simulink model "external_memory_test"  (R2020b)
settings: Solver=FixedStepDiscrete  StartTime=0.0  StopTime=80  RelTol=1e-3
InitFcn:
  | Feature_Width = 64;
  | Feature_Height = 64;
  | Weight_Width = 3;
  | Weight_Height = 3;
  | external_memory_test_init;
values from neighbouring files (symbols this model uses):
  Burst_Length = Feature_Weight_Length    [external_memory_test_init.m]
  byPass = 1    [external_memory_test_init.m]
  Conv_Padding = 0    [external_memory_test_init.m]
  Conv_Stride = 1    [external_memory_test_init.m]
  DDR_Depth = Weight_Length + Feature_Length + outFeature_Length    [external_memory_test_init.m]
  ddrInitData = single((rand(1,DDR_Depth)))    [external_memory_test_init.m]
  Duty_Cycle = 0.5    [external_memory_test_init.m]
  Feature_Area = Feature_Width * Feature_Height    [external_memory_test_init.m]
  Feature_Length = Phase_In * Feature_Area    [external_memory_test_init.m]
  inChannel = 3    [external_memory_test_init.m]
  outChannel = 2    [external_memory_test_init.m]
  outFeature_Length = outFeature_Width * outFeature_Height * Phase_Out    [external_memory_test_init.m]
  Pool_Stride = 2    [external_memory_test_init.m]
  Pool_Width = 2    [external_memory_test_init.m]
  Tc = 1    [external_memory_test_init.m]
  Ti = 1    [external_memory_test_init.m]
  To = 1    [external_memory_test_init.m]
  Tr = 1    [external_memory_test_init.m]
  Weight_Length = Phase_In * Weight_Area * Phase_Out    [external_memory_test_init.m]
undefined symbols (not defined in the file or in its folder): Conv_Step, Pool_Step, sigbuilder_block
libraries: hdlsllib x85, simulink x44, visionhdlutilities x16
(part 3 of 6)

== system external_memory_test/DUT/2DConvPE V1.0/Subsystem2 ==
  In1 : Inport
  Bus Selector : BusSelector  OutputSignals=signal1,signal2,signal3,signal4,signal5,signal6,signal7,signal8,signal9,signal10,signal11,signal12,signal13,signal14,signal15
  Weight_Length : Outport
  Weight_Area : Outport  Port=2
  Weight_Width : Outport  Port=3
  Weight_Height : Outport  Port=4
  Feature_Length : Outport  Port=5
  Feature_Area : Outport  Port=6
  Feature_Width : Outport  Port=7
  Feature_Height : Outport  Port=8
  outFeature_Length : Outport  Port=9
  outFeature_Area : Outport  Port=10
  outFeature_Width : Outport  Port=11
  outFeature_Height : Outport  Port=12
  Conv_Step : Outport  Port=13
  inChannel : Outport  Port=14
  outChannel : Outport  Port=15
  wires:
  In1/1 -> Bus Selector/1
  Bus Selector/1 -> Weight_Length/1  "<signal1>"
  Bus Selector/2 -> Weight_Area/1  "<signal2>"
  Bus Selector/3 -> Weight_Width/1  "<signal3>"
  Bus Selector/4 -> Weight_Height/1  "<signal4>"
  Bus Selector/5 -> Feature_Length/1  "<signal5>"
  Bus Selector/6 -> Feature_Area/1  "<signal6>"
  Bus Selector/7 -> Feature_Width/1  "<signal7>"
  Bus Selector/8 -> Feature_Height/1  "<signal8>"
  Bus Selector/9 -> outFeature_Length/1  "<signal9>"
  Bus Selector/10 -> outFeature_Area/1  "<signal10>"
  Bus Selector/11 -> outFeature_Width/1  "<signal11>"
  Bus Selector/12 -> outFeature_Height/1  "<signal12>"
  Bus Selector/13 -> Conv_Step/1  "<signal13>"
  Bus Selector/14 -> inChannel/1  "<signal14>"
  Bus Selector/15 -> outChannel/1  "<signal15>"

== system external_memory_test/DUT/2DConvPE V1.0/Window Selector ==
  In1 : Inport
  valid : Inport  Port=2
  step : Inport  Port=3
  Add : Sum  Inputs=+-
  Compare To Zero : simulink/Logic and Bit Operations/Compare To Zero  relop===  OutDataTypeStr=boolean
  Constant : Constant  OutDataTypeStr=uint32
  Delay : Delay
  Delay1 : Delay  DelayLength=3
  Delay2 : Delay  DelayLength=1
  Delay3 : Delay  DelayLength=1
  Delay4 : Delay  DelayLength=1
  Logical Operator : Logic  Operator=NOT  AllPortsSameDT=off  OutDataTypeStr=boolean
  Logical Operator1 : Logic  Operator=OR  AllPortsSameDT=off  OutDataTypeStr=boolean
  Logical Operator2 : Logic  AllPortsSameDT=off  OutDataTypeStr=boolean
  Relational Operator : RelationalOperator  OutDataTypeStr=boolean  RndMeth=Nearest
  Selector1 : Selector  InputPortWidth=3  IndexOptions=Index vector (dialog)  Indices=[1]  OutputSizes=1
  Selector2 : Selector  InputPortWidth=3  IndexOptions=Index vector (dialog)  Indices=[2]  OutputSizes=1
  Selector3 : Selector  InputPortWidth=3  IndexOptions=Index vector (dialog)  Indices=[3]  OutputSizes=1
  Selector4 : Selector  InputPortWidth=3  IndexOptions=Index vector (dialog)  Indices=[1]  OutputSizes=1
  Selector5 : Selector  InputPortWidth=3  IndexOptions=Index vector (dialog)  Indices=[2]  OutputSizes=1
  Selector6 : Selector  InputPortWidth=3  IndexOptions=Index vector (dialog)  Indices=[3]  OutputSizes=1
  Selector7 : Selector  InputPortWidth=3  IndexOptions=Index vector (dialog)  Indices=[1]  OutputSizes=1
  Selector8 : Selector  InputPortWidth=3  IndexOptions=Index vector (dialog)  Indices=[2]  OutputSizes=1
  Selector9 : Selector  InputPortWidth=3  IndexOptions=Index vector (dialog)  Indices=[3]  OutputSizes=1
  Step Counter : hdlsllib/Sources/HDL Counter  CountType=Free running  CountInit=0  CountStep=1  CountMax=2^15  CountFromType=Initial value  CountFrom=0  CountResetPort=on  CountLoadPort=off  CountEnbPort=on  CountDirPort=off  CountDataType=Unsigned  CountWordLen=32  CountFracLen=0  CountSampTime=1
  Out1 : Outport
  Out2 : Outport  Port=2
  Out3 : Outport  Port=3
  Out4 : Outport  Port=4
  Out5 : Outport  Port=5
  Out6 : Outport  Port=6
  Out7 : Outport  Port=7
  Out8 : Outport  Port=8
  Out9 : Outport  Port=9
  Valid : Outport  Port=10
  wires:
  Selector2/1 -> Out2/1
  In1/1 -> Delay2/1, Delay1/1, Delay/1
  Selector1/1 -> Out1/1
  Selector3/1 -> Out3/1
  Selector8/1 -> Out5/1
  Selector9/1 -> Out6/1
  Selector7/1 -> Out4/1
  Delay/1 -> Selector9/1, Selector8/1, Selector7/1
  Selector5/1 -> Out8/1
  Selector6/1 -> Out9/1
  Selector4/1 -> Out7/1
  Delay1/1 -> Selector6/1, Selector5/1, Selector4/1
  Relational Operator/1 -> Logical Operator1/1
  Constant/1 -> Add/2
  Logical Operator2/1 -> Valid/1
  Compare To Zero/1 -> Logical Operator2/1
  Logical Operator1/1 -> Step Counter/1
  Logical Operator/1 -> Logical Operator1/2
  Delay4/1 -> Add/1
  Step Counter/1 -> Compare To Zero/1, Relational Operator/1
  Delay3/1 -> Logical Operator2/2, Step Counter/2, Logical Operator/1
  Add/1 -> Relational Operator/2
  Delay2/1 -> Selector3/1, Selector2/1, Selector1/1
  valid/1 -> Delay3/1
  step/1 -> Delay4/1

== system external_memory_test/DUT/2DConvPE V1.1/Adder Tree ==
  In1 : Inport
  In2 : Inport  Port=2
  In3 : Inport  Port=3
  In4 : Inport  Port=4
  In5 : Inport  Port=5
  In6 : Inport  Port=6
  In7 : Inport  Port=7
  In8 : Inport  Port=8
  In9 : Inport  Port=9
  validIn : Inport  Port=10
  Add{,1..6,10} (8 alike) : Sum
  Delay{1..9,35} (10 alike) : Delay  DelayLength=1
  Out1 : Outport
  validOut : Outport  Port=2
  wires:
  Add/1 -> Add4/1
  Add4/1 -> Add6/1
  Add10/1 -> Out1/1
  Add3/1 -> Add5/2
  Add2/1 -> Add5/1
  Add1/1 -> Add4/2
  Add6/1 -> Add10/1
  Add5/1 -> Add6/2
  Delay35/1 -> Add/1
  Delay1/1 -> Add/2
  Delay3/1 -> Add1/1
  Delay2/1 -> Add1/2
  Delay5/1 -> Add2/1
  Delay4/1 -> Add2/2
  Delay7/1 -> Add3/1
  Delay6/1 -> Add3/2
  In9/1 -> Delay8/1
  Delay8/1 -> Add10/2
  In8/1 -> Delay6/1
  In7/1 -> Delay7/1
  In6/1 -> Delay4/1
  In5/1 -> Delay5/1
  In4/1 -> Delay2/1
  In3/1 -> Delay3/1
  In2/1 -> Delay1/1
  In1/1 -> Delay35/1
  validIn/1 -> Delay9/1
  Delay9/1 -> validOut/1

== system external_memory_test/DUT/2DConvPE V1.1/Address Logic ==
  note: W/R_Address_Gen
  In1 : Inport
  In2 : Inport  Port=2
  " " : Subsystem
  Add : Sum  Inputs=+-
  Compare To Constant : simulink/Logic and Bit Operations/Compare To Constant  relop===  const=0  OutDataTypeStr=boolean
  Constant : Constant  OutDataTypeStr=uint32
  Delay : Delay  DelayLength=1
  Logical Operator1 : Logic  AllPortsSameDT=off  OutDataTypeStr=boolean
  Logical Operator2 : Logic  Operator=NOT  AllPortsSameDT=off  OutDataTypeStr=boolean
  Relational Operator : RelationalOperator  OutDataTypeStr=boolean  RndMeth=Simplest
  Weight_Counter : hdlsllib/Sources/HDL Counter  CountType=Free running  CountInit=0  CountStep=1  CountMax=2^15  CountFromType=Initial value  CountFrom=0  CountResetPort=on  CountLoadPort=off  CountEnbPort=on  CountDirPort=off  CountDataType=Unsigned  CountWordLen=32  CountFracLen=0  CountSampTime=1
  Weight_Interation_Counter : hdlsllib/Sources/HDL Counter  CountType=Free running  CountInit=0  CountStep=1  CountMax=2^15  CountFromType=Initial value  CountFrom=0  CountResetPort=on  CountLoadPort=off  CountEnbPort=on  CountDirPort=off  CountDataType=Unsigned  CountWordLen=32  CountFracLen=0  CountSampTime=1
  W : Outport
  Write_en : Outport  Port=2
  R : Outport  Port=3
  wires:
  Weight_Counter/1 -> " "/1(In1), Relational Operator/1
  Compare To Constant/1 -> Write_en/1, " "/2(In2)
  Delay/1 -> Logical Operator1/2, Logical Operator2/1, Weight_Counter/2
  Weight_Interation_Counter/1 -> Compare To Constant/1
  Constant/1 -> Add/2
  Logical Operator2/1 -> Weight_Interation_Counter/1
  " "/1(W) -> W/1
  Logical Operator1/1 -> Weight_Counter/1
  Relational Operator/1 -> Weight_Interation_Counter/2, Logical Operator1/1
  Add/1 -> Relational Operator/2
  In1/1 -> Delay/1
  In2/1 -> Add/1
  " "/2(R) -> R/1

== system external_memory_test/DUT/2DConvPE V1.1/AddressGen ==
  enb : Inport
  PhaseOut_Count : Inport  Port=2
  outFeature_Area : Inport  Port=3
  ADD : Sum
  Constant1 : Constant  Value=0  OutDataTypeStr=uint32  SampleTime=-1
  Constant2 : Constant  OutDataTypeStr=uint32  SampleTime=-1
  Minus : Sum  Inputs=+-
  OutAddress_Counter : hdlsllib/Sources/HDL Counter  CountType=Free running  CountInit=0  CountStep=1  CountMax=2^15  CountFromType=Initial value  CountFrom=0  CountResetPort=on  CountLoadPort=off  CountEnbPort=on  CountDirPort=off  CountDataType=Unsigned  CountWordLen=32  CountFracLen=0  CountSampTime=1
  Product : Product
  Relational Operator : RelationalOperator  OutDataTypeStr=boolean  RndMeth=Nearest
  Switch : Switch  Criteria=u2 ~= 0
  OutAdddess : Outport
  wires:
  Constant1/1 -> Switch/1
  Switch/1 -> Product/2
  OutAddress_Counter/1 -> Relational Operator/1, ADD/2
  outFeature_Area/1 -> Product/1, Minus/1
  Relational Operator/1 -> OutAddress_Counter/1
  Constant2/1 -> Minus/2
  Product/1 -> ADD/1
  ADD/1 -> OutAdddess/1
  Minus/1 -> Relational Operator/2
  enb/1 -> Switch/2, OutAddress_Counter/2
  PhaseOut_Count/1 -> Switch/3

== system external_memory_test/DUT/2DConvPE V1.1/LIne Buffer ==
  Stream_In : Inport
  Stream_Valid : Inport  Port=2
  Weight_Width : Inport  Port=3
  Feature_Area : Inport  Port=4
  Feature_Width : Inport  Port=5
  Feature_Height : Inport  Port=6
  Delay2 : Delay  DelayLength=1
  Line Buffer : Subsystem
  OutValidGen : Subsystem
  Terminator : Terminator
  pixel : Outport
  valid : Outport  Port=2
  wires:
  Feature_Area/1 -> Line Buffer/3(Feature_Area)
  Feature_Height/1 -> OutValidGen/3(Feature_Height)
  Line Buffer/3(shftEnable) -> Terminator/1
  Stream_In/1 -> Line Buffer/1(Stream_In)
  Line Buffer/1(pixel) -> Delay2/1
  Line Buffer/2(ctrl) -> OutValidGen/1(In1)
  Feature_Width/1 -> Line Buffer/4(Feature_Width)
  Stream_Valid/1 -> Line Buffer/2(Stream_Valid)
  Weight_Width/1 -> OutValidGen/2(Weight_Width)
  OutValidGen/1(valid) -> valid/1
  Delay2/1 -> pixel/1

== system external_memory_test/DUT/2DConvPE V1.1/MaxPooling ==
  Stream_In : Inport
  Stream_Valid : Inport  Port=2
  ByPass : Inport  Port=3
  step : Inport  Port=4
  Window_Width : Inport  Port=5
  Feature_Area : Inport  Port=6
  Feature_Width : Inport  Port=7
  Feature_Height : Inport  Port=8
  Comparator : Subsystem
  Constant : Constant  Value=0  OutDataTypeStr=int32
  Delay{,1..6,36} (8 alike) : Delay  DelayLength=1
  Line Buffer1 : Subsystem
  OutValidGen : Subsystem
  Switch : Switch  Criteria=u2 > Threshold
  Switch1 : Switch  Criteria=u2 > Threshold
  Terminator1 : Terminator
  dataSwitch : Switch  Criteria=u2 > Threshold
  validSwitch : Switch  Criteria=u2 > Threshold
  window Selector : Subsystem
  outdata : Outport
  Valid : Outport  Port=2
  wires:
  window Selector/3(Out3) -> Delay3/1
  OutValidGen/1(Out1) -> window Selector/2(valid)
  Feature_Width/1 -> Line Buffer1/4(Feature_Width)
  Line Buffer1/3(shftEnable) -> Terminator1/1
  Window_Width/1 -> OutValidGen/2(Window_Width)
  window Selector/5(Valid) -> Delay5/1
  window Selector/1(Out1) -> Delay/1
  Line Buffer1/1(pixel) -> Delay2/1
  Line Buffer1/2(ctrl) -> OutValidGen/1(ctrl)
  window Selector/2(Out2) -> Delay6/1
  window Selector/4(Out4) -> Delay4/1
  Feature_Area/1 -> Line Buffer1/3(Feature_Area)
  Feature_Height/1 -> OutValidGen/3(Feature_Height)
  step/1 -> window Selector/3(step)
  Delay1/1 -> validSwitch/1, Switch1/3
  Comparator/1(Out1) -> dataSwitch/3
  Delay36/1 -> dataSwitch/1, Switch/3
  ByPass/1 -> validSwitch/2, dataSwitch/2, Switch1/2, Switch/2
  dataSwitch/1 -> outdata/1
  validSwitch/1 -> Valid/1
  Constant/1 -> Switch1/1, Switch/1
  Switch/1 -> Line Buffer1/1(Stream_In)
  Switch1/1 -> Line Buffer1/2(Stream_Valid)
  Comparator/2(outvalid) -> validSwitch/3
  Stream_In/1 -> Delay36/1
  Stream_Valid/1 -> Delay1/1
  Delay2/1 -> window Selector/1(pixel)
  Delay/1 -> Comparator/1(In1)
  Delay5/1 -> Comparator/5(Valid)
  Delay4/1 -> Comparator/4(In4)
  Delay3/1 -> Comparator/3(In3)
  Delay6/1 -> Comparator/2(In2)

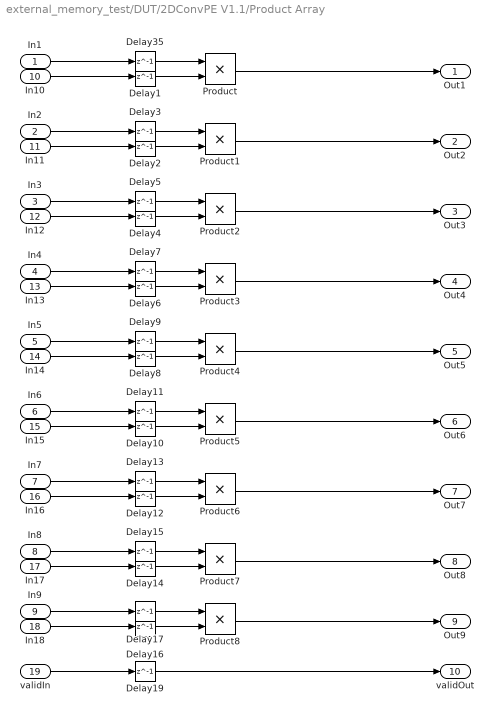
== system external_memory_test/DUT/2DConvPE V1.1/Product Array ==
  In1 : Inport
  In2 : Inport  Port=2
  In3 : Inport  Port=3
  In4 : Inport  Port=4
  In5 : Inport  Port=5
  In6 : Inport  Port=6
  In7 : Inport  Port=7
  In8 : Inport  Port=8
  In9 : Inport  Port=9
  In10 : Inport  Port=10
  In11 : Inport  Port=11
  In12 : Inport  Port=12
  In13 : Inport  Port=13
  In14 : Inport  Port=14
  In15 : Inport  Port=15
  In16 : Inport  Port=16
  In17 : Inport  Port=17
  In18 : Inport  Port=18
  validIn : Inport  Port=19
  Delay{1..17,19,35} (19 alike) : Delay  DelayLength=1
  Product{,1..8} (9 alike) : Product
  Out1 : Outport
  Out2 : Outport  Port=2
  Out3 : Outport  Port=3
  Out4 : Outport  Port=4
  Out5 : Outport  Port=5
  Out6 : Outport  Port=6
  Out7 : Outport  Port=7
  Out8 : Outport  Port=8
  Out9 : Outport  Port=9
  validOut : Outport  Port=10
  wires:
  Product/1 -> Out1/1
  In4/1 -> Delay7/1
  Product4/1 -> Out5/1
  In8/1 -> Delay15/1
  In17/1 -> Delay14/1
  In9/1 -> Delay17/1
  In12/1 -> Delay4/1
  In7/1 -> Delay13/1
  In1/1 -> Delay35/1
  In13/1 -> Delay6/1
  Product1/1 -> Out2/1
  In16/1 -> Delay12/1
  In10/1 -> Delay1/1
  In14/1 -> Delay8/1
  In18/1 -> Delay16/1
  Product8/1 -> Out9/1
  Product7/1 -> Out8/1
  In6/1 -> Delay11/1
  In2/1 -> Delay3/1
  In11/1 -> Delay2/1
  In15/1 -> Delay10/1
  In5/1 -> Delay9/1
  In3/1 -> Delay5/1
  Product3/1 -> Out4/1
  Product2/1 -> Out3/1
  Product5/1 -> Out6/1
  Product6/1 -> Out7/1
  validIn/1 -> Delay19/1
  Delay1/1 -> Product/2
  Delay35/1 -> Product/1
  Delay3/1 -> Product1/1
  Delay2/1 -> Product1/2
  Delay5/1 -> Product2/1
  Delay4/1 -> Product2/2
  Delay7/1 -> Product3/1
  Delay6/1 -> Product3/2
  Delay8/1 -> Product4/2
  Delay9/1 -> Product4/1
  Delay11/1 -> Product5/1
  Delay10/1 -> Product5/2
  Delay13/1 -> Product6/1
  Delay12/1 -> Product6/2
  Delay14/1 -> Product7/2
  Delay15/1 -> Product7/1
  Delay17/1 -> Product8/1
  Delay16/1 -> Product8/2
  Delay19/1 -> validOut/1

== system external_memory_test/DUT/2DConvPE V1.1/ReLU ==
  data_in : Inport
  validIn : Inport  Port=2
  byPass : Inport  Port=3
  Compare To Zero : simulink/Logic and Bit Operations/Compare To Zero  relop=>  OutDataTypeStr=boolean
  Constant : Constant  Value=0  OutDataTypeStr=int32
  Delay1 : Delay  DelayLength=1
  Delay36 : Delay  DelayLength=1
  Switch : Switch  Criteria=u2 > Threshold
  Switch1 : Switch  Criteria=u2 > Threshold
  data_ReLU : Outport
  valildOut : Outport  Port=2
  wires:
  Constant/1 -> Switch/3
  Delay36/1 -> Switch1/1, Switch/1, Compare To Zero/1
  Compare To Zero/1 -> Switch/2
  Switch/1 -> Switch1/3
  byPass/1 -> Switch1/2
  Switch1/1 -> data_ReLU/1
  Delay1/1 -> valildOut/1
  data_in/1 -> Delay36/1
  validIn/1 -> Delay1/1

== system external_memory_test/DUT/2DConvPE V1.1/Subsystem ==
  In1 : Inport
  Bus Selector : BusSelector  OutputSignals=signal1,signal2
  pool_step : Outport
  pool_Width : Outport  Port=2
  wires:
  Bus Selector/2 -> pool_Width/1  "<signal2>"
  Bus Selector/1 -> pool_step/1  "<signal1>"
  In1/1 -> Bus Selector/1

== system external_memory_test/DUT/2DConvPE V1.1/Subsystem2 ==
  In1 : Inport
  Bus Selector : BusSelector  OutputSignals=signal1,signal2,signal3,signal4,signal5,signal6,signal7,signal8,signal9,signal10,signal11,signal12,signal13,signal14,signal15
  Weight_Length : Outport
  Weight_Area : Outport  Port=2
  Weight_Width : Outport  Port=3
  Weight_Height : Outport  Port=4
  Feature_Length : Outport  Port=5
  Feature_Area : Outport  Port=6
  Feature_Width : Outport  Port=7
  Feature_Height : Outport  Port=8
  outFeature_Length : Outport  Port=9
  outFeature_Area : Outport  Port=10
  outFeature_Width : Outport  Port=11
  outFeature_Height : Outport  Port=12
  Conv_Step : Outport  Port=13
  inChannel : Outport  Port=14
  outChannel : Outport  Port=15
  wires:
  In1/1 -> Bus Selector/1
  Bus Selector/1 -> Weight_Length/1  "<signal1>"
  Bus Selector/2 -> Weight_Area/1  "<signal2>"
  Bus Selector/3 -> Weight_Width/1  "<signal3>"
  Bus Selector/4 -> Weight_Height/1  "<signal4>"
  Bus Selector/5 -> Feature_Length/1  "<signal5>"
  Bus Selector/6 -> Feature_Area/1  "<signal6>"
  Bus Selector/7 -> Feature_Width/1  "<signal7>"
  Bus Selector/8 -> Feature_Height/1  "<signal8>"
  Bus Selector/9 -> outFeature_Length/1  "<signal9>"
  Bus Selector/10 -> outFeature_Area/1  "<signal10>"
  Bus Selector/11 -> outFeature_Width/1  "<signal11>"
  Bus Selector/12 -> outFeature_Height/1  "<signal12>"
  Bus Selector/13 -> Conv_Step/1  "<signal13>"
  Bus Selector/14 -> inChannel/1  "<signal14>"
  Bus Selector/15 -> outChannel/1  "<signal15>"

== system external_memory_test/DUT/2DConvPE V1.1/Window Selector ==
  In1 : Inport
  valid : Inport  Port=2
  step : Inport  Port=3
  Add : Sum  Inputs=+-
  Compare To Zero : simulink/Logic and Bit Operations/Compare To Zero  relop===  OutDataTypeStr=boolean
  Constant : Constant  OutDataTypeStr=uint32
  Delay : Delay
  Delay1 : Delay  DelayLength=3
  Delay2 : Delay  DelayLength=1
  Delay3 : Delay  DelayLength=1
  Delay4 : Delay  DelayLength=1
  Logical Operator : Logic  Operator=NOT  AllPortsSameDT=off  OutDataTypeStr=boolean
  Logical Operator1 : Logic  Operator=OR  AllPortsSameDT=off  OutDataTypeStr=boolean
  Logical Operator2 : Logic  AllPortsSameDT=off  OutDataTypeStr=boolean
  Relational Operator : RelationalOperator  OutDataTypeStr=boolean  RndMeth=Nearest
  Selector1 : Selector  InputPortWidth=3  IndexOptions=Index vector (dialog)  Indices=[1]  OutputSizes=1
  Selector2 : Selector  InputPortWidth=3  IndexOptions=Index vector (dialog)  Indices=[2]  OutputSizes=1
  Selector3 : Selector  InputPortWidth=3  IndexOptions=Index vector (dialog)  Indices=[3]  OutputSizes=1
  Selector4 : Selector  InputPortWidth=3  IndexOptions=Index vector (dialog)  Indices=[1]  OutputSizes=1
  Selector5 : Selector  InputPortWidth=3  IndexOptions=Index vector (dialog)  Indices=[2]  OutputSizes=1
  Selector6 : Selector  InputPortWidth=3  IndexOptions=Index vector (dialog)  Indices=[3]  OutputSizes=1
  Selector7 : Selector  InputPortWidth=3  IndexOptions=Index vector (dialog)  Indices=[1]  OutputSizes=1
  Selector8 : Selector  InputPortWidth=3  IndexOptions=Index vector (dialog)  Indices=[2]  OutputSizes=1
  Selector9 : Selector  InputPortWidth=3  IndexOptions=Index vector (dialog)  Indices=[3]  OutputSizes=1
  Step Counter : hdlsllib/Sources/HDL Counter  CountType=Free running  CountInit=0  CountStep=1  CountMax=2^15  CountFromType=Initial value  CountFrom=0  CountResetPort=on  CountLoadPort=off  CountEnbPort=on  CountDirPort=off  CountDataType=Unsigned  CountWordLen=32  CountFracLen=0  CountSampTime=1
  Out1 : Outport
  Out2 : Outport  Port=2
  Out3 : Outport  Port=3
  Out4 : Outport  Port=4
  Out5 : Outport  Port=5
  Out6 : Outport  Port=6
  Out7 : Outport  Port=7
  Out8 : Outport  Port=8
  Out9 : Outport  Port=9
  Valid : Outport  Port=10
  wires:
  Selector2/1 -> Out2/1
  In1/1 -> Delay2/1, Delay1/1, Delay/1
  Selector1/1 -> Out1/1
  Selector3/1 -> Out3/1
  Selector8/1 -> Out5/1
  Selector9/1 -> Out6/1
  Selector7/1 -> Out4/1
  Delay/1 -> Selector9/1, Selector8/1, Selector7/1
  Selector5/1 -> Out8/1
  Selector6/1 -> Out9/1
  Selector4/1 -> Out7/1
  Delay1/1 -> Selector6/1, Selector5/1, Selector4/1
  Relational Operator/1 -> Logical Operator1/1
  Constant/1 -> Add/2
  Logical Operator2/1 -> Valid/1
  Compare To Zero/1 -> Logical Operator2/1
  Logical Operator1/1 -> Step Counter/1
  Logical Operator/1 -> Logical Operator1/2
  Delay4/1 -> Add/1
  Step Counter/1 -> Compare To Zero/1, Relational Operator/1
  Delay3/1 -> Logical Operator2/2, Step Counter/2, Logical Operator/1
  Add/1 -> Relational Operator/2
  Delay2/1 -> Selector3/1, Selector2/1, Selector1/1
  valid/1 -> Delay3/1
  step/1 -> Delay4/1

== system external_memory_test/DUT/2DConvPE V1.2/Adder Tree ==
  In1 : Inport
  In2 : Inport  Port=2
  In3 : Inport  Port=3
  In4 : Inport  Port=4
  In5 : Inport  Port=5
  In6 : Inport  Port=6
  In7 : Inport  Port=7
  In8 : Inport  Port=8
  In9 : Inport  Port=9
  validIn : Inport  Port=10
  Add{,1..6,10} (8 alike) : Sum
  Delay{1..9,35} (10 alike) : Delay  DelayLength=1
  Out1 : Outport
  validOut : Outport  Port=2
  wires:
  Add/1 -> Add4/1
  Add4/1 -> Add6/1
  Add10/1 -> Out1/1
  Add3/1 -> Add5/2
  Add2/1 -> Add5/1
  Add1/1 -> Add4/2
  Add6/1 -> Add10/1
  Add5/1 -> Add6/2
  Delay35/1 -> Add/1
  Delay1/1 -> Add/2
  Delay3/1 -> Add1/1
  Delay2/1 -> Add1/2
  Delay5/1 -> Add2/1
  Delay4/1 -> Add2/2
  Delay7/1 -> Add3/1
  Delay6/1 -> Add3/2
  In9/1 -> Delay8/1
  Delay8/1 -> Add10/2
  In8/1 -> Delay6/1
  In7/1 -> Delay7/1
  In6/1 -> Delay4/1
  In5/1 -> Delay5/1
  In4/1 -> Delay2/1
  In3/1 -> Delay3/1
  In2/1 -> Delay1/1
  In1/1 -> Delay35/1
  validIn/1 -> Delay9/1
  Delay9/1 -> validOut/1

== system external_memory_test/DUT/2DConvPE V1.2/Address Logic ==
  note: W/R_Address_Gen
  In1 : Inport
  In2 : Inport  Port=2
  " " : Subsystem
  Add : Sum  Inputs=+-
  Compare To Constant : simulink/Logic and Bit Operations/Compare To Constant  relop===  const=0  OutDataTypeStr=boolean
  Constant : Constant  OutDataTypeStr=uint32
  Delay : Delay  DelayLength=1
  Logical Operator1 : Logic  AllPortsSameDT=off  OutDataTypeStr=boolean
  Logical Operator2 : Logic  Operator=NOT  AllPortsSameDT=off  OutDataTypeStr=boolean
  Relational Operator : RelationalOperator  OutDataTypeStr=boolean  RndMeth=Simplest
  Weight_Counter : hdlsllib/Sources/HDL Counter  CountType=Free running  CountInit=0  CountStep=1  CountMax=2^15  CountFromType=Initial value  CountFrom=0  CountResetPort=on  CountLoadPort=off  CountEnbPort=on  CountDirPort=off  CountDataType=Unsigned  CountWordLen=32  CountFracLen=0  CountSampTime=1
  Weight_Interation_Counter : hdlsllib/Sources/HDL Counter  CountType=Free running  CountInit=0  CountStep=1  CountMax=2^15  CountFromType=Initial value  CountFrom=0  CountResetPort=on  CountLoadPort=off  CountEnbPort=on  CountDirPort=off  CountDataType=Unsigned  CountWordLen=32  CountFracLen=0  CountSampTime=1
  W : Outport
  Write_en : Outport  Port=2
  R : Outport  Port=3
  wires:
  Weight_Counter/1 -> " "/1(In1), Relational Operator/1
  Compare To Constant/1 -> Write_en/1, " "/2(In2)
  Delay/1 -> Logical Operator1/2, Logical Operator2/1, Weight_Counter/2
  Weight_Interation_Counter/1 -> Compare To Constant/1
  Constant/1 -> Add/2
  Logical Operator2/1 -> Weight_Interation_Counter/1
  " "/1(W) -> W/1
  Logical Operator1/1 -> Weight_Counter/1
  Relational Operator/1 -> Weight_Interation_Counter/2, Logical Operator1/1
  Add/1 -> Relational Operator/2
  In1/1 -> Delay/1
  In2/1 -> Add/1
  " "/2(R) -> R/1

== system external_memory_test/DUT/2DConvPE V1.2/AddressGen ==
  enb : Inport
  PhaseOut_Count : Inport  Port=2
  outFeature_Area : Inport  Port=3
  ADD : Sum
  Constant1 : Constant  Value=0  OutDataTypeStr=uint32  SampleTime=-1
  Constant2 : Constant  OutDataTypeStr=uint32  SampleTime=-1
  Minus : Sum  Inputs=+-
  OutAddress_Counter : hdlsllib/Sources/HDL Counter  CountType=Free running  CountInit=0  CountStep=1  CountMax=2^15  CountFromType=Initial value  CountFrom=0  CountResetPort=on  CountLoadPort=off  CountEnbPort=on  CountDirPort=off  CountDataType=Unsigned  CountWordLen=32  CountFracLen=0  CountSampTime=1
  Product : Product
  Relational Operator : RelationalOperator  OutDataTypeStr=boolean  RndMeth=Nearest
  Switch : Switch  Criteria=u2 ~= 0
  OutAdddess : Outport
  wires:
  Constant1/1 -> Switch/1
  Switch/1 -> Product/2
  OutAddress_Counter/1 -> Relational Operator/1, ADD/2
  outFeature_Area/1 -> Product/1, Minus/1
  Relational Operator/1 -> OutAddress_Counter/1
  Constant2/1 -> Minus/2
  Product/1 -> ADD/1
  ADD/1 -> OutAdddess/1
  Minus/1 -> Relational Operator/2
  enb/1 -> Switch/2, OutAddress_Counter/2
  PhaseOut_Count/1 -> Switch/3

== system external_memory_test/DUT/2DConvPE V1.2/LIne Buffer ==
  Stream_In : Inport
  Stream_Valid : Inport  Port=2
  Weight_Width : Inport  Port=3
  Feature_Area : Inport  Port=4
  Feature_Width : Inport  Port=5
  Feature_Height : Inport  Port=6
  Delay2 : Delay  DelayLength=1
  Line Buffer : Subsystem
  OutValidGen : Subsystem
  Terminator : Terminator
  pixel : Outport
  valid : Outport  Port=2
  wires:
  Feature_Area/1 -> Line Buffer/3(Feature_Area)
  Feature_Height/1 -> OutValidGen/3(Feature_Height)
  Line Buffer/3(shftEnable) -> Terminator/1
  Stream_In/1 -> Line Buffer/1(Stream_In)
  Line Buffer/1(pixel) -> Delay2/1
  Line Buffer/2(ctrl) -> OutValidGen/1(In1)
  Feature_Width/1 -> Line Buffer/4(Feature_Width)
  Stream_Valid/1 -> Line Buffer/2(Stream_Valid)
  Weight_Width/1 -> OutValidGen/2(Weight_Width)
  OutValidGen/1(valid) -> valid/1
  Delay2/1 -> pixel/1

== system external_memory_test/DUT/2DConvPE V1.2/MaxPooling ==
  Stream_In : Inport
  Stream_Valid : Inport  Port=2
  ByPass : Inport  Port=3
  step : Inport  Port=4
  Window_Width : Inport  Port=5
  Feature_Area : Inport  Port=6
  Feature_Width : Inport  Port=7
  Feature_Height : Inport  Port=8
  Comparator : Subsystem
  Constant : Constant  Value=0  OutDataTypeStr=int32
  Delay{,1..6,36} (8 alike) : Delay  DelayLength=1
  Line Buffer1 : Subsystem
  OutValidGen : Subsystem
  Switch : Switch  Criteria=u2 > Threshold
  Switch1 : Switch  Criteria=u2 > Threshold
  Terminator1 : Terminator
  dataSwitch : Switch  Criteria=u2 > Threshold
  validSwitch : Switch  Criteria=u2 > Threshold
  window Selector : Subsystem
  outdata : Outport
  Valid : Outport  Port=2
  wires:
  window Selector/3(Out3) -> Delay3/1
  OutValidGen/1(Out1) -> window Selector/2(valid)
  Feature_Width/1 -> Line Buffer1/4(Feature_Width)
  Line Buffer1/3(shftEnable) -> Terminator1/1
  Window_Width/1 -> OutValidGen/2(Window_Width)
  window Selector/5(Valid) -> Delay5/1
  window Selector/1(Out1) -> Delay/1
  Line Buffer1/1(pixel) -> Delay2/1
  Line Buffer1/2(ctrl) -> OutValidGen/1(ctrl)
  window Selector/2(Out2) -> Delay6/1
  window Selector/4(Out4) -> Delay4/1
  Feature_Area/1 -> Line Buffer1/3(Feature_Area)
  Feature_Height/1 -> OutValidGen/3(Feature_Height)
  step/1 -> window Selector/3(step)
  Delay1/1 -> validSwitch/1, Switch1/3
  Comparator/1(Out1) -> dataSwitch/3
  Delay36/1 -> dataSwitch/1, Switch/3
  ByPass/1 -> validSwitch/2, dataSwitch/2, Switch1/2, Switch/2
  dataSwitch/1 -> outdata/1
  validSwitch/1 -> Valid/1
  Constant/1 -> Switch1/1, Switch/1
  Switch/1 -> Line Buffer1/1(Stream_In)
  Switch1/1 -> Line Buffer1/2(Stream_Valid)
  Comparator/2(outvalid) -> validSwitch/3
  Stream_In/1 -> Delay36/1
  Stream_Valid/1 -> Delay1/1
  Delay2/1 -> window Selector/1(pixel)
  Delay/1 -> Comparator/1(In1)
  Delay5/1 -> Comparator/5(Valid)
  Delay4/1 -> Comparator/4(In4)
  Delay3/1 -> Comparator/3(In3)
  Delay6/1 -> Comparator/2(In2)

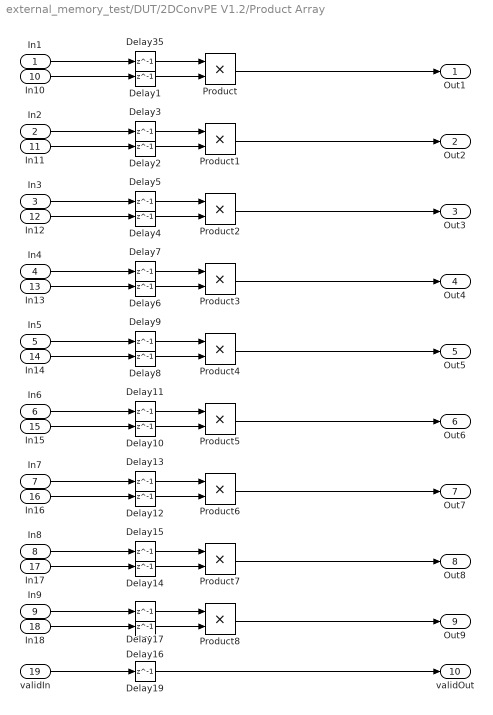
== system external_memory_test/DUT/2DConvPE V1.2/Product Array ==
  In1 : Inport
  In2 : Inport  Port=2
  In3 : Inport  Port=3
  In4 : Inport  Port=4
  In5 : Inport  Port=5
  In6 : Inport  Port=6
  In7 : Inport  Port=7
  In8 : Inport  Port=8
  In9 : Inport  Port=9
  In10 : Inport  Port=10
  In11 : Inport  Port=11
  In12 : Inport  Port=12
  In13 : Inport  Port=13
  In14 : Inport  Port=14
  In15 : Inport  Port=15
  In16 : Inport  Port=16
  In17 : Inport  Port=17
  In18 : Inport  Port=18
  validIn : Inport  Port=19
  Delay{1..17,19,35} (19 alike) : Delay  DelayLength=1
  Product{,1..8} (9 alike) : Product
  Out1 : Outport
  Out2 : Outport  Port=2
  Out3 : Outport  Port=3
  Out4 : Outport  Port=4
  Out5 : Outport  Port=5
  Out6 : Outport  Port=6
  Out7 : Outport  Port=7
  Out8 : Outport  Port=8
  Out9 : Outport  Port=9
  validOut : Outport  Port=10
  wires:
  Product/1 -> Out1/1
  In4/1 -> Delay7/1
  Product4/1 -> Out5/1
  In8/1 -> Delay15/1
  In17/1 -> Delay14/1
  In9/1 -> Delay17/1
  In12/1 -> Delay4/1
  In7/1 -> Delay13/1
  In1/1 -> Delay35/1
  In13/1 -> Delay6/1
  Product1/1 -> Out2/1
  In16/1 -> Delay12/1
  In10/1 -> Delay1/1
  In14/1 -> Delay8/1
  In18/1 -> Delay16/1
  Product8/1 -> Out9/1
  Product7/1 -> Out8/1
  In6/1 -> Delay11/1
  In2/1 -> Delay3/1
  In11/1 -> Delay2/1
  In15/1 -> Delay10/1
  In5/1 -> Delay9/1
  In3/1 -> Delay5/1
  Product3/1 -> Out4/1
  Product2/1 -> Out3/1
  Product5/1 -> Out6/1
  Product6/1 -> Out7/1
  validIn/1 -> Delay19/1
  Delay1/1 -> Product/2
  Delay35/1 -> Product/1
  Delay3/1 -> Product1/1
  Delay2/1 -> Product1/2
  Delay5/1 -> Product2/1
  Delay4/1 -> Product2/2
  Delay7/1 -> Product3/1
  Delay6/1 -> Product3/2
  Delay8/1 -> Product4/2
  Delay9/1 -> Product4/1
  Delay11/1 -> Product5/1
  Delay10/1 -> Product5/2
  Delay13/1 -> Product6/1
  Delay12/1 -> Product6/2
  Delay14/1 -> Product7/2
  Delay15/1 -> Product7/1
  Delay17/1 -> Product8/1
  Delay16/1 -> Product8/2
  Delay19/1 -> validOut/1

== system external_memory_test/DUT/2DConvPE V1.2/ReLU ==
  data_in : Inport
  validIn : Inport  Port=2
  byPass : Inport  Port=3
  Compare To Zero : simulink/Logic and Bit Operations/Compare To Zero  relop=>  OutDataTypeStr=boolean
  Constant : Constant  Value=0  OutDataTypeStr=int32
  Delay1 : Delay  DelayLength=1
  Delay36 : Delay  DelayLength=1
  Switch : Switch  Criteria=u2 > Threshold
  Switch1 : Switch  Criteria=u2 > Threshold
  data_ReLU : Outport
  valildOut : Outport  Port=2
  wires:
  Constant/1 -> Switch/3
  Delay36/1 -> Switch1/1, Switch/1, Compare To Zero/1
  Compare To Zero/1 -> Switch/2
  Switch/1 -> Switch1/3
  byPass/1 -> Switch1/2
  Switch1/1 -> data_ReLU/1
  Delay1/1 -> valildOut/1
  data_in/1 -> Delay36/1
  validIn/1 -> Delay1/1

== system external_memory_test/DUT/2DConvPE V1.2/Subsystem ==
  In1 : Inport
  Bus Selector : BusSelector  OutputSignals=signal1,signal2
  pool_step : Outport
  pool_Width : Outport  Port=2
  wires:
  Bus Selector/2 -> pool_Width/1  "<signal2>"
  Bus Selector/1 -> pool_step/1  "<signal1>"
  In1/1 -> Bus Selector/1

== system external_memory_test/DUT/2DConvPE V1.2/Subsystem2 ==
  In1 : Inport
  Bus Selector : BusSelector  OutputSignals=signal1,signal2,signal3,signal4,signal5,signal6,signal7,signal8,signal9,signal10,signal11,signal12,signal13,signal14,signal15
  Weight_Length : Outport
  Weight_Area : Outport  Port=2
  Weight_Width : Outport  Port=3
  Weight_Height : Outport  Port=4
  Feature_Length : Outport  Port=5
  Feature_Area : Outport  Port=6
  Feature_Width : Outport  Port=7
  Feature_Height : Outport  Port=8
  outFeature_Length : Outport  Port=9
  outFeature_Area : Outport  Port=10
  outFeature_Width : Outport  Port=11
  outFeature_Height : Outport  Port=12
  Conv_Step : Outport  Port=13
  inChannel : Outport  Port=14
  outChannel : Outport  Port=15
  wires:
  In1/1 -> Bus Selector/1
  Bus Selector/1 -> Weight_Length/1  "<signal1>"
  Bus Selector/2 -> Weight_Area/1  "<signal2>"
  Bus Selector/3 -> Weight_Width/1  "<signal3>"
  Bus Selector/4 -> Weight_Height/1  "<signal4>"
  Bus Selector/5 -> Feature_Length/1  "<signal5>"
  Bus Selector/6 -> Feature_Area/1  "<signal6>"
  Bus Selector/7 -> Feature_Width/1  "<signal7>"
  Bus Selector/8 -> Feature_Height/1  "<signal8>"
  Bus Selector/9 -> outFeature_Length/1  "<signal9>"
  Bus Selector/10 -> outFeature_Area/1  "<signal10>"
  Bus Selector/11 -> outFeature_Width/1  "<signal11>"
  Bus Selector/12 -> outFeature_Height/1  "<signal12>"
  Bus Selector/13 -> Conv_Step/1  "<signal13>"
  Bus Selector/14 -> inChannel/1  "<signal14>"
  Bus Selector/15 -> outChannel/1  "<signal15>"

== system external_memory_test/DUT/2DConvPE V1.2/Window Selector ==
  In1 : Inport
  valid : Inport  Port=2
  step : Inport  Port=3
  Add : Sum  Inputs=+-
  Compare To Zero : simulink/Logic and Bit Operations/Compare To Zero  relop===  OutDataTypeStr=boolean
  Constant : Constant  OutDataTypeStr=uint32
  Delay : Delay
  Delay1 : Delay  DelayLength=3
  Delay2 : Delay  DelayLength=1
  Delay3 : Delay  DelayLength=1
  Delay4 : Delay  DelayLength=1
  Logical Operator : Logic  Operator=NOT  AllPortsSameDT=off  OutDataTypeStr=boolean
  Logical Operator1 : Logic  Operator=OR  AllPortsSameDT=off  OutDataTypeStr=boolean
  Logical Operator2 : Logic  AllPortsSameDT=off  OutDataTypeStr=boolean
  Relational Operator : RelationalOperator  OutDataTypeStr=boolean  RndMeth=Nearest
  Selector1 : Selector  InputPortWidth=3  IndexOptions=Index vector (dialog)  Indices=[1]  OutputSizes=1
  Selector2 : Selector  InputPortWidth=3  IndexOptions=Index vector (dialog)  Indices=[2]  OutputSizes=1
  Selector3 : Selector  InputPortWidth=3  IndexOptions=Index vector (dialog)  Indices=[3]  OutputSizes=1
  Selector4 : Selector  InputPortWidth=3  IndexOptions=Index vector (dialog)  Indices=[1]  OutputSizes=1
  Selector5 : Selector  InputPortWidth=3  IndexOptions=Index vector (dialog)  Indices=[2]  OutputSizes=1
  Selector6 : Selector  InputPortWidth=3  IndexOptions=Index vector (dialog)  Indices=[3]  OutputSizes=1
  Selector7 : Selector  InputPortWidth=3  IndexOptions=Index vector (dialog)  Indices=[1]  OutputSizes=1
  Selector8 : Selector  InputPortWidth=3  IndexOptions=Index vector (dialog)  Indices=[2]  OutputSizes=1
  Selector9 : Selector  InputPortWidth=3  IndexOptions=Index vector (dialog)  Indices=[3]  OutputSizes=1
  Step Counter : hdlsllib/Sources/HDL Counter  CountType=Free running  CountInit=0  CountStep=1  CountMax=2^15  CountFromType=Initial value  CountFrom=0  CountResetPort=on  CountLoadPort=off  CountEnbPort=on  CountDirPort=off  CountDataType=Unsigned  CountWordLen=32  CountFracLen=0  CountSampTime=1
  Out1 : Outport
  Out2 : Outport  Port=2
  Out3 : Outport  Port=3
  Out4 : Outport  Port=4
  Out5 : Outport  Port=5
  Out6 : Outport  Port=6
  Out7 : Outport  Port=7
  Out8 : Outport  Port=8
  Out9 : Outport  Port=9
  Valid : Outport  Port=10
  wires:
  Selector2/1 -> Out2/1
  In1/1 -> Delay2/1, Delay1/1, Delay/1
  Selector1/1 -> Out1/1
  Selector3/1 -> Out3/1
  Selector8/1 -> Out5/1
  Selector9/1 -> Out6/1
  Selector7/1 -> Out4/1
  Delay/1 -> Selector9/1, Selector8/1, Selector7/1
  Selector5/1 -> Out8/1
  Selector6/1 -> Out9/1
  Selector4/1 -> Out7/1
  Delay1/1 -> Selector6/1, Selector5/1, Selector4/1
  Relational Operator/1 -> Logical Operator1/1
  Constant/1 -> Add/2
  Logical Operator2/1 -> Valid/1
  Compare To Zero/1 -> Logical Operator2/1
  Logical Operator1/1 -> Step Counter/1
  Logical Operator/1 -> Logical Operator1/2
  Delay4/1 -> Add/1
  Step Counter/1 -> Compare To Zero/1, Relational Operator/1
  Delay3/1 -> Logical Operator2/2, Step Counter/2, Logical Operator/1
  Add/1 -> Relational Operator/2
  Delay2/1 -> Selector3/1, Selector2/1, Selector1/1
  valid/1 -> Delay3/1
  step/1 -> Delay4/1

== system external_memory_test/DUT/2DConvPE V1.3/Adder Tree ==
  In1 : Inport
  In2 : Inport  Port=2
  In3 : Inport  Port=3
  In4 : Inport  Port=4
  In5 : Inport  Port=5
  In6 : Inport  Port=6
  In7 : Inport  Port=7
  In8 : Inport  Port=8
  In9 : Inport  Port=9
  validIn : Inport  Port=10
  Add{,1..6,10} (8 alike) : Sum
  Delay{1..9,35} (10 alike) : Delay  DelayLength=1
  Out1 : Outport
  validOut : Outport  Port=2
  wires:
  Add/1 -> Add4/1
  Add4/1 -> Add6/1
  Add10/1 -> Out1/1
  Add3/1 -> Add5/2
  Add2/1 -> Add5/1
  Add1/1 -> Add4/2
  Add6/1 -> Add10/1
  Add5/1 -> Add6/2
  Delay35/1 -> Add/1
  Delay1/1 -> Add/2
  Delay3/1 -> Add1/1
  Delay2/1 -> Add1/2
  Delay5/1 -> Add2/1
  Delay4/1 -> Add2/2
  Delay7/1 -> Add3/1
  Delay6/1 -> Add3/2
  In9/1 -> Delay8/1
  Delay8/1 -> Add10/2
  In8/1 -> Delay6/1
  In7/1 -> Delay7/1
  In6/1 -> Delay4/1
  In5/1 -> Delay5/1
  In4/1 -> Delay2/1
  In3/1 -> Delay3/1
  In2/1 -> Delay1/1
  In1/1 -> Delay35/1
  validIn/1 -> Delay9/1
  Delay9/1 -> validOut/1

== system external_memory_test/DUT/2DConvPE V1.3/Address Logic ==
  note: W/R_Address_Gen
  In1 : Inport
  In2 : Inport  Port=2
  " " : Subsystem
  Add : Sum  Inputs=+-
  Compare To Constant : simulink/Logic and Bit Operations/Compare To Constant  relop===  const=0  OutDataTypeStr=boolean
  Constant : Constant  OutDataTypeStr=uint32
  Delay : Delay  DelayLength=1
  Logical Operator1 : Logic  AllPortsSameDT=off  OutDataTypeStr=boolean
  Logical Operator2 : Logic  Operator=NOT  AllPortsSameDT=off  OutDataTypeStr=boolean
  Relational Operator : RelationalOperator  OutDataTypeStr=boolean  RndMeth=Simplest
  Weight_Counter : hdlsllib/Sources/HDL Counter  CountType=Free running  CountInit=0  CountStep=1  CountMax=2^15  CountFromType=Initial value  CountFrom=0  CountResetPort=on  CountLoadPort=off  CountEnbPort=on  CountDirPort=off  CountDataType=Unsigned  CountWordLen=32  CountFracLen=0  CountSampTime=1
  Weight_Interation_Counter : hdlsllib/Sources/HDL Counter  CountType=Free running  CountInit=0  CountStep=1  CountMax=2^15  CountFromType=Initial value  CountFrom=0  CountResetPort=on  CountLoadPort=off  CountEnbPort=on  CountDirPort=off  CountDataType=Unsigned  CountWordLen=32  CountFracLen=0  CountSampTime=1
  W : Outport
  Write_en : Outport  Port=2
  R : Outport  Port=3
  wires:
  Weight_Counter/1 -> " "/1(In1), Relational Operator/1
  Compare To Constant/1 -> Write_en/1, " "/2(In2)
  Delay/1 -> Logical Operator1/2, Logical Operator2/1, Weight_Counter/2
  Weight_Interation_Counter/1 -> Compare To Constant/1
  Constant/1 -> Add/2
  Logical Operator2/1 -> Weight_Interation_Counter/1
  " "/1(W) -> W/1
  Logical Operator1/1 -> Weight_Counter/1
  Relational Operator/1 -> Weight_Interation_Counter/2, Logical Operator1/1
  Add/1 -> Relational Operator/2
  In1/1 -> Delay/1
  In2/1 -> Add/1
  " "/2(R) -> R/1

== system external_memory_test/DUT/2DConvPE V1.3/AddressGen ==
  enb : Inport
  PhaseOut_Count : Inport  Port=2
  outFeature_Area : Inport  Port=3
  ADD : Sum
  Constant1 : Constant  Value=0  OutDataTypeStr=uint32  SampleTime=-1
  Constant2 : Constant  OutDataTypeStr=uint32  SampleTime=-1
  Minus : Sum  Inputs=+-
  OutAddress_Counter : hdlsllib/Sources/HDL Counter  CountType=Free running  CountInit=0  CountStep=1  CountMax=2^15  CountFromType=Initial value  CountFrom=0  CountResetPort=on  CountLoadPort=off  CountEnbPort=on  CountDirPort=off  CountDataType=Unsigned  CountWordLen=32  CountFracLen=0  CountSampTime=1
  Product : Product
  Relational Operator : RelationalOperator  OutDataTypeStr=boolean  RndMeth=Nearest
  Switch : Switch  Criteria=u2 ~= 0
  OutAdddess : Outport
  wires:
  Constant1/1 -> Switch/1
  Switch/1 -> Product/2
  OutAddress_Counter/1 -> Relational Operator/1, ADD/2
  outFeature_Area/1 -> Product/1, Minus/1
  Relational Operator/1 -> OutAddress_Counter/1
  Constant2/1 -> Minus/2
  Product/1 -> ADD/1
  ADD/1 -> OutAdddess/1
  Minus/1 -> Relational Operator/2
  enb/1 -> Switch/2, OutAddress_Counter/2
  PhaseOut_Count/1 -> Switch/3

== system external_memory_test/DUT/2DConvPE V1.3/LIne Buffer ==
  Stream_In : Inport
  Stream_Valid : Inport  Port=2
  Weight_Width : Inport  Port=3
  Feature_Area : Inport  Port=4
  Feature_Width : Inport  Port=5
  Feature_Height : Inport  Port=6
  Delay2 : Delay  DelayLength=1
  Line Buffer : Subsystem
  OutValidGen : Subsystem
  Terminator : Terminator
  pixel : Outport
  valid : Outport  Port=2
  wires:
  Feature_Area/1 -> Line Buffer/3(Feature_Area)
  Feature_Height/1 -> OutValidGen/3(Feature_Height)
  Line Buffer/3(shftEnable) -> Terminator/1
  Stream_In/1 -> Line Buffer/1(Stream_In)
  Line Buffer/1(pixel) -> Delay2/1
  Line Buffer/2(ctrl) -> OutValidGen/1(In1)
  Feature_Width/1 -> Line Buffer/4(Feature_Width)
  Stream_Valid/1 -> Line Buffer/2(Stream_Valid)
  Weight_Width/1 -> OutValidGen/2(Weight_Width)
  OutValidGen/1(valid) -> valid/1
  Delay2/1 -> pixel/1

== system external_memory_test/DUT/2DConvPE V1.3/MaxPooling ==
  Stream_In : Inport
  Stream_Valid : Inport  Port=2
  ByPass : Inport  Port=3
  step : Inport  Port=4
  Window_Width : Inport  Port=5
  Feature_Area : Inport  Port=6
  Feature_Width : Inport  Port=7
  Feature_Height : Inport  Port=8
  Comparator : Subsystem
  Constant : Constant  Value=0  OutDataTypeStr=int32
  Delay{,1..6,36} (8 alike) : Delay  DelayLength=1
  Line Buffer1 : Subsystem
  OutValidGen : Subsystem
  Switch : Switch  Criteria=u2 > Threshold
  Switch1 : Switch  Criteria=u2 > Threshold
  Terminator1 : Terminator
  dataSwitch : Switch  Criteria=u2 > Threshold
  validSwitch : Switch  Criteria=u2 > Threshold
  window Selector : Subsystem
  outdata : Outport
  Valid : Outport  Port=2
  wires:
  window Selector/3(Out3) -> Delay3/1
  OutValidGen/1(Out1) -> window Selector/2(valid)
  Feature_Width/1 -> Line Buffer1/4(Feature_Width)
  Line Buffer1/3(shftEnable) -> Terminator1/1
  Window_Width/1 -> OutValidGen/2(Window_Width)
  window Selector/5(Valid) -> Delay5/1
  window Selector/1(Out1) -> Delay/1
  Line Buffer1/1(pixel) -> Delay2/1
  Line Buffer1/2(ctrl) -> OutValidGen/1(ctrl)
  window Selector/2(Out2) -> Delay6/1
  window Selector/4(Out4) -> Delay4/1
  Feature_Area/1 -> Line Buffer1/3(Feature_Area)
  Feature_Height/1 -> OutValidGen/3(Feature_Height)
  step/1 -> window Selector/3(step)
  Delay1/1 -> validSwitch/1, Switch1/3
  Comparator/1(Out1) -> dataSwitch/3
  Delay36/1 -> dataSwitch/1, Switch/3
  ByPass/1 -> validSwitch/2, dataSwitch/2, Switch1/2, Switch/2
  dataSwitch/1 -> outdata/1
  validSwitch/1 -> Valid/1
  Constant/1 -> Switch1/1, Switch/1
  Switch/1 -> Line Buffer1/1(Stream_In)
  Switch1/1 -> Line Buffer1/2(Stream_Valid)
  Comparator/2(outvalid) -> validSwitch/3
  Stream_In/1 -> Delay36/1
  Stream_Valid/1 -> Delay1/1
  Delay2/1 -> window Selector/1(pixel)
  Delay/1 -> Comparator/1(In1)
  Delay5/1 -> Comparator/5(Valid)
  Delay4/1 -> Comparator/4(In4)
  Delay3/1 -> Comparator/3(In3)
  Delay6/1 -> Comparator/2(In2)

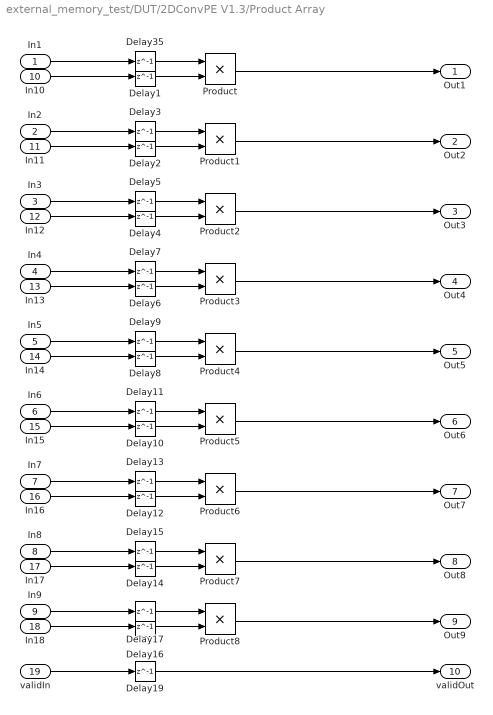
== system external_memory_test/DUT/2DConvPE V1.3/Product Array ==
  In1 : Inport
  In2 : Inport  Port=2
  In3 : Inport  Port=3
  In4 : Inport  Port=4
  In5 : Inport  Port=5
  In6 : Inport  Port=6
  In7 : Inport  Port=7
  In8 : Inport  Port=8
  In9 : Inport  Port=9
  In10 : Inport  Port=10
  In11 : Inport  Port=11
  In12 : Inport  Port=12
  In13 : Inport  Port=13
  In14 : Inport  Port=14
  In15 : Inport  Port=15
  In16 : Inport  Port=16
  In17 : Inport  Port=17
  In18 : Inport  Port=18
  validIn : Inport  Port=19
  Delay{1..17,19,35} (19 alike) : Delay  DelayLength=1
  Product{,1..8} (9 alike) : Product
  Out1 : Outport
  Out2 : Outport  Port=2
  Out3 : Outport  Port=3
  Out4 : Outport  Port=4
  Out5 : Outport  Port=5
  Out6 : Outport  Port=6
  Out7 : Outport  Port=7
  Out8 : Outport  Port=8
  Out9 : Outport  Port=9
  validOut : Outport  Port=10
  wires:
  Product/1 -> Out1/1
  In4/1 -> Delay7/1
  Product4/1 -> Out5/1
  In8/1 -> Delay15/1
  In17/1 -> Delay14/1
  In9/1 -> Delay17/1
  In12/1 -> Delay4/1
  In7/1 -> Delay13/1
  In1/1 -> Delay35/1
  In13/1 -> Delay6/1
  Product1/1 -> Out2/1
  In16/1 -> Delay12/1
  In10/1 -> Delay1/1
  In14/1 -> Delay8/1
  In18/1 -> Delay16/1
  Product8/1 -> Out9/1
  Product7/1 -> Out8/1
  In6/1 -> Delay11/1
  In2/1 -> Delay3/1
  In11/1 -> Delay2/1
  In15/1 -> Delay10/1
  In5/1 -> Delay9/1
  In3/1 -> Delay5/1
  Product3/1 -> Out4/1
  Product2/1 -> Out3/1
  Product5/1 -> Out6/1
  Product6/1 -> Out7/1
  validIn/1 -> Delay19/1
  Delay1/1 -> Product/2
  Delay35/1 -> Product/1
  Delay3/1 -> Product1/1
  Delay2/1 -> Product1/2
  Delay5/1 -> Product2/1
  Delay4/1 -> Product2/2
  Delay7/1 -> Product3/1
  Delay6/1 -> Product3/2
  Delay8/1 -> Product4/2
  Delay9/1 -> Product4/1
  Delay11/1 -> Product5/1
  Delay10/1 -> Product5/2
  Delay13/1 -> Product6/1
  Delay12/1 -> Product6/2
  Delay14/1 -> Product7/2
  Delay15/1 -> Product7/1
  Delay17/1 -> Product8/1
  Delay16/1 -> Product8/2
  Delay19/1 -> validOut/1

== system external_memory_test/DUT/2DConvPE V1.3/ReLU ==
  data_in : Inport
  validIn : Inport  Port=2
  byPass : Inport  Port=3
  Compare To Zero : simulink/Logic and Bit Operations/Compare To Zero  relop=>  OutDataTypeStr=boolean
  Constant : Constant  Value=0  OutDataTypeStr=int32
  Delay1 : Delay  DelayLength=1
  Delay36 : Delay  DelayLength=1
  Switch : Switch  Criteria=u2 > Threshold
  Switch1 : Switch  Criteria=u2 > Threshold
  data_ReLU : Outport
  valildOut : Outport  Port=2
  wires:
  Constant/1 -> Switch/3
  Delay36/1 -> Switch1/1, Switch/1, Compare To Zero/1
  Compare To Zero/1 -> Switch/2
  Switch/1 -> Switch1/3
  byPass/1 -> Switch1/2
  Switch1/1 -> data_ReLU/1
  Delay1/1 -> valildOut/1
  data_in/1 -> Delay36/1
  validIn/1 -> Delay1/1

== system external_memory_test/DUT/2DConvPE V1.3/Subsystem ==
  In1 : Inport
  Bus Selector : BusSelector  OutputSignals=signal1,signal2
  pool_step : Outport
  pool_Width : Outport  Port=2
  wires:
  Bus Selector/2 -> pool_Width/1  "<signal2>"
  Bus Selector/1 -> pool_step/1  "<signal1>"
  In1/1 -> Bus Selector/1

== system external_memory_test/DUT/2DConvPE V1.3/Subsystem2 ==
  In1 : Inport
  Bus Selector : BusSelector  OutputSignals=signal1,signal2,signal3,signal4,signal5,signal6,signal7,signal8,signal9,signal10,signal11,signal12,signal13,signal14,signal15
  Weight_Length : Outport
  Weight_Area : Outport  Port=2
  Weight_Width : Outport  Port=3
  Weight_Height : Outport  Port=4
  Feature_Length : Outport  Port=5
  Feature_Area : Outport  Port=6
  Feature_Width : Outport  Port=7
  Feature_Height : Outport  Port=8
  outFeature_Length : Outport  Port=9
  outFeature_Area : Outport  Port=10
  outFeature_Width : Outport  Port=11
  outFeature_Height : Outport  Port=12
  Conv_Step : Outport  Port=13
  inChannel : Outport  Port=14
  outChannel : Outport  Port=15
  wires:
  In1/1 -> Bus Selector/1
  Bus Selector/1 -> Weight_Length/1  "<signal1>"
  Bus Selector/2 -> Weight_Area/1  "<signal2>"
  Bus Selector/3 -> Weight_Width/1  "<signal3>"
  Bus Selector/4 -> Weight_Height/1  "<signal4>"
  Bus Selector/5 -> Feature_Length/1  "<signal5>"
  Bus Selector/6 -> Feature_Area/1  "<signal6>"
  Bus Selector/7 -> Feature_Width/1  "<signal7>"
  Bus Selector/8 -> Feature_Height/1  "<signal8>"
  Bus Selector/9 -> outFeature_Length/1  "<signal9>"
  Bus Selector/10 -> outFeature_Area/1  "<signal10>"
  Bus Selector/11 -> outFeature_Width/1  "<signal11>"
  Bus Selector/12 -> outFeature_Height/1  "<signal12>"
  Bus Selector/13 -> Conv_Step/1  "<signal13>"
  Bus Selector/14 -> inChannel/1  "<signal14>"
  Bus Selector/15 -> outChannel/1  "<signal15>"
